simulink model "ObstacleAvoidance"  (R2023a)
settings: Solver=ode4  StartTime=0.0  StopTime=T_stop  RelTol=1e-4  AbsTol=1e-4
StartFcn:
  | close all;
  | rho_cfrp = 6.32;
  | Ts = 1e-4;
  | Tsc = Ts;
undefined symbols (not defined in the file): k_air, Kii, Kiw, Kpi, Kpw, l_bat, miu_air, Opacity, p, planedepth, planex, planey, pr_air, T_stop, Temp, Vdc, X, xrot, Y, yrot, Z, zrot
libraries: sm_lib x356, nesl_utility x78, fl_lib x65, ee_lib x17, slpidlib x8, eeBldcCurrentController x4, eePwmGenerator x4, eeGeneralControl x4, test_library x4, batteryecm_lib x1
(part 8 of 8)

== system ObstacleAvoidance/Quadcopter/propeller4/Sensing w a1/Hall sensor/Subsystem ==
  theta : Inport
  Trigonometric Function : Trigonometry  Operator=sincos
  Trigonometric Function2 : Trigonometry  Operator=atan2
  mech->elec : Gain  Gain=p
  rad->deg : Gain  Gain=180/pi  SaturateOnIntegerOverflow=on  OutDataTypeStr=Inherit: Same as input  ParamDataTypeStr=Inherit: Same as input
  deg : Outport  VectorParamsAs1DForOutWhenUnconnected=off
  wires:
  Trigonometric Function2/1 -> rad->deg/1
  Trigonometric Function/1 -> Trigonometric Function2/1
  theta/1 -> mech->elec/1
  rad->deg/1 -> deg/1
  Trigonometric Function/2 -> Trigonometric Function2/2
  mech->elec/1 -> Trigonometric Function/1

== matlab function ObstacleAvoidance/Manuver Controller/attitude planner ==
  data: des_pos input; des_vel input; des_acc input; des_yaw input; pos input; vel input; pitch_des output; roll_des output; yaw_des output
function [pitch_des,roll_des,yaw_des] = attitude_planner(des_pos,des_vel,des_acc,des_yaw,pos,vel)
%PID parameter value
kp_1 = 3.5;
kp_2 =3.5;
kd_1 = 2;
kd_2 = 2;

% obtain the desired state
acc_1_des = des_acc(1)+kd_1*(des_vel(1)-vel(1))+kp_1*(des_pos(1)-pos(1));
acc_2_des = des_acc(2)+kd_2*(des_vel(2)-vel(2))+kp_2*(des_pos(2)-pos(2));

pitch_des   = (1/9.81)*(acc_1_des*sin(des_yaw)-acc_2_des*cos(des_yaw));
roll_des = (1/9.81)*(acc_1_des*cos(des_yaw)+acc_2_des*sin(des_yaw));
yaw_des = des_yaw;

if des_pos(1) == 0 && des_pos(2) == 0 && des_pos(3) == 5 && des_vel(1) == 0 && des_vel(2) == 0 && des_vel(3) == 0
    pitch_des = 0;
    roll_des = 0;
    yaw_des = 0;
end
end

== matlab function ObstacleAvoidance/Manuver Controller/helix_traj_generator ==
  data: t input; des_pos output; des_vel output; des_acc output; des_yaw output; stepSize input; endTime input
function [des_pos,des_vel,des_acc,des_yaw]  = traj_generator(t,stepSize,endTime)
%% Titile
% This is the function used to calculate the optimum trajectory of given
% waypoints as well as the fixed time step t. The output of the function
% would be the desired state of quadcopter, which includes the target
% position, velocity and acceleration. This function should be used in
% sequence with attitude planner to give desired pitch, roll and yaw angle
% of quadcopter.
% Written by Tian Wang
% 14/08/2019

%% main
% r = 2.5;
% x =zeros(1,13);
% y = x;
% z = x;
% for t = (0:1:12)
%     x(t+1) = r*cos(t);
%     y(t+1) = r*sin(t);
%     z(t+1) = 3+5/12*t;
% end
% 
% waypoints = [x;y;z];
waypoints =[2.50000000000000,1.35075576467035,-1.04036709136786,-2.47498124150111,-1.63410905215903,0.709155463658066,2.40042571662592,1.88475563585826,-0.363750084521534,-2.27782565471169,-2.09767882269113,0.0110642449701270,2.10963489683123;0,2.10367746201974,2.27324356706420,0.352800020149668,-1.89200623826982,-2.39731068665785,-0.698538745497315,1.64246649679697,2.47339561655845,1.03029621310439,-1.36005277722342,-2.49997551637676,-1.34143229500109;3,3.41666666666667,3.83333333333333,4.25000000000000,4.66666666666667,5.08333333333333,5.50000000000000,5.91666666666667,6.33333333333333,6.75000000000000,7.16666666666667,7.58333333333333,8];
traj_step = size(waypoints);
timespot = linspace(0,endTime,(traj_step(2)));
pp = spline(timespot, waypoints);
% if(t == 0)
%     des_pos = waypoints(:,1);
% else
    des_pos = ppval(pp,t);
% end
des_vel = (ppval(pp,t+stepSize)-ppval(pp,t))./stepSize;
des_acc = zeros(3,1);
des_yaw = 0;



    

end

== matlab function ObstacleAvoidance/Manuver Controller/Astar Alog ==
  data: y input; waypoints output; t input; des_pos output double size=[3 1]; des_vel output double size=[3 1]; des_acc output double size=[3 1]; des_yaw output double; stepSize input; endTime input
function [waypoints,des_pos,des_vel,des_acc,des_yaw]  = traj_generator(y,t,stepSize,endTime)
%% Titile
% This is the function used to calculate the optimum trajectory of given
% waypoints as well as the fixed time step t. The output of the function
% would be the desired state of quadcopter, which includes the target
% position, velocity and acceleration. This function should be used in
% sequence with attitude planner to give desired pitch, roll and yaw angle
% of quadcopter.
% Written by Tian Wang
% 14/08/2019

%% main
 waypoints = [1.50000000000000,1.50000000000000,2.50000000000000,3.50000000000000,4.50000000000000,5.50000000000000,6.50000000000000,6.50000000000000,6.50000000000000,7.50000000000000,8.50000000000000,8.50000000000000,8.50000000000000,8.50000000000000,8.50000000000000,8.50000000000000,8.50000000000000,8.50000000000000;-5.50000000000000,-5.50000000000000,-5.50000000000000,-5.50000000000000,-5.50000000000000,-5.50000000000000,-5.50000000000000,-4.50000000000000,-3.50000000000000,-3.50000000000000,-3.50000000000000,-5.50000000000000,-7.50000000000000,-9.50000000000000,-9.50000000000000,-9.50000000000000,-9.50000000000000,-9.50000000000000;6,4,4,4,4,4,4,4,4,4,4,4,4,4,4,4,4,4];
% waypoints = [1.50000000000000,2.50000000000000,3.50000000000000,4.50000000000000,5.50000000000000,6.50000000000000,6.50000000000000,6.50000000000000,6.50000000000000,6.50000000000000,5.50000000000000,4.50000000000000,3.50000000000000,2.50000000000000,1.50000000000000,0.500000000000000,0.500000000000000;-5.50000000000000,-5.50000000000000,-5.50000000000000,-5.50000000000000,-5.50000000000000,-5.50000000000000,-6.50000000000000,-7.50000000000000,-8.50000000000000,-9.50000000000000,-9.50000000000000,-9.50000000000000,-9.50000000000000,-9.50000000000000,-9.50000000000000,-9.50000000000000,-9.50000000000000;5,5,5,5,5,5,5,5,5,5,5,5,5,5,5,5,2.50000000000000];
% waypoints = [1.5 1.5 1.5;-5.5 -5.5 -5.5; 5 5 5];
traj_step = size(waypoints);
timespot = linspace(0,endTime,(traj_step(2)));
pp = spline(timespot, waypoints);
if y == 0
    des_pos = ppval(pp,t);
    des_vel = (ppval(pp,t+stepSize)-ppval(pp,t))./stepSize;
else 
    des_pos = zeros(3,1);
    des_pos(3) =5; 
    des_vel = zeros(3,1);
end
des_acc = zeros(3,1);
des_yaw = 0;





end

== matlab function ObstacleAvoidance/Manuver Controller/waypoint_traj_generator2 ==
  data: t input; des_pos output; des_vel output; des_acc output; des_yaw output; stepSize input; endTime input
function [des_pos,des_vel,des_acc,des_yaw]  = traj_generator(t,stepSize,endTime)
%% Titile
% This is the function used to calculate the optimum trajectory of given
% waypoints as well as the fixed time step t. The output of the function
% would be the desired state of quadcopter, which includes the target
% position, velocity and acceleration. This function should be used in
% sequence with attitude planner to give desired pitch, roll and yaw angle
% of quadcopter.
% Written by Tian Wang
% 14/08/2019

%% main
% r = 2.5;
% x =zeros(1,13);
% y = x;
% z = x;
% for t = (0:1:12)
%     x(t+1) = r*cos(t);
%     y(t+1) = r*sin(t);
%     z(t+1) = 3+5/12*t;
% end
% 
% waypoints = [x;y;z];
% waypoints =[2.50000000000000,1.35075576467035,-1.04036709136786,-2.47498124150111,-1.63410905215903,0.709155463658066,2.40042571662592,1.88475563585826,-0.363750084521534,-2.27782565471169,-2.09767882269113,0.0110642449701270,2.10963489683123;0,2.10367746201974,2.27324356706420,0.352800020149668,-1.89200623826982,-2.39731068665785,-0.698538745497315,1.64246649679697,2.47339561655845,1.03029621310439,-1.36005277722342,-2.49997551637676,-1.34143229500109;3,3.41666666666667,3.83333333333333,4.25000000000000,4.66666666666667,5.08333333333333,5.50000000000000,5.91666666666667,6.33333333333333,6.75000000000000,7.16666666666667,7.58333333333333,8];
waypoints = [ 0 0 6;
                          1 2 5;
                          2 -2 4;
                          4 -4 7]';
traj_step = size(waypoints);
timespot = linspace(0,endTime,(traj_step(2)));
pp = spline(timespot, waypoints);
% if(t == 0)
%     des_pos = waypoints(:,1);
% else
    des_pos = ppval(pp,t);
% end
des_vel = (ppval(pp,t+stepSize)-ppval(pp,t))./stepSize;
des_acc = zeros(3,1);
des_yaw = 0;



    

end

== matlab function ObstacleAvoidance/Manuver Controller/MATLAB Function ==
  data: pitch input; y output; roll input
function y = fcn(pitch,roll)
y=0;
    if abs(pitch) > 30/180*pi
        y = 1;
    elseif abs(roll) > 30/180*pi
        y = 1;
    else
        y=0;
    end

end
